simulink model "voltage_to_fahrenheit_system"  (R2020b)
settings: Solver=ode45  StartTime=0.0  StopTime=220  RelTol=1e-3  EnableMultiTasking=on
libraries: simulink x1
settings Model: Creator=USER  LastModifiedBy=USER
settings DataIOCC: LimitDataPoints=on  SaveFormat=Array  ReturnWorkspaceOutputs=off
settings OptimizationCC: LifeSpan=inf
settings DebuggingCC: SFUnexpectedBacktrackingDiag=warning  SFNoUnconditionalDefaultTransitionDiag=warning  SFExecutionAtInitializationDiag=none  ArithmeticOperatorsInVariantConditions=warning
settings HardwareCC: ProdBitPerPointer=32  ProdBitPerSizeT=32  ProdBitPerPtrDiffT=32  ProdLargestAtomicFloat=None  ProdIntDivRoundTo=Undefined  ProdEndianess=Unspecified  ProdWordSize=32  ProdHWDeviceType=32-bit Generic
settings ModelReferenceCC: PropagateSignalLabelsOutOfModel=off
settings SFSimCC: SimUseLocalCustomCode=off  CustomCodeUndefinedFunction=UseInterfaceOnly
settings RTWCC: RTWUseLocalCustomCode=off
settings CodeAppCC: StateflowObjectComments=on
settings GRTTargetCC: TargetLangStandard=C89/C90 (ANSI)
settings ConfigComp: CovMetricSettings=dw  CovSaveCumulativeToWorkspaceVar=on  CovSaveSingleToWorkspaceVar=on  CovExternalEMLEnable=off

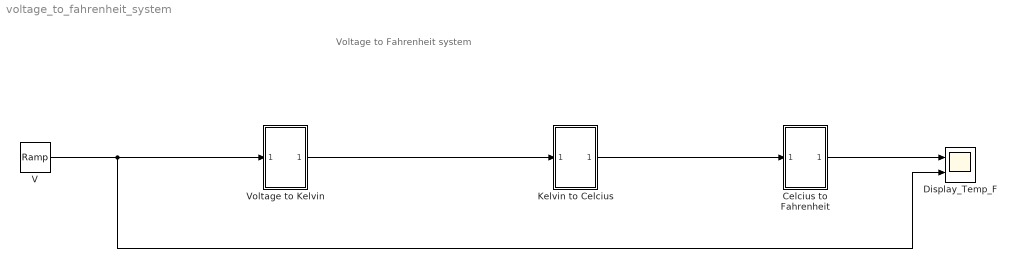
== system voltage_to_fahrenheit_system ==
  note: Voltage to Fahrenheit system
  Celcius to Fahrenheit : Subsystem
  Display_Temp_F : Scope  NumInputPorts=2
  Kelvin to Celcius : Subsystem
  V : simulink/Sources/Ramp  slope=20  start=0  InitialOutput=0
  Voltage to Kelvin : Subsystem
  wires:
  V/1 -> Display_Temp_F/2, Voltage to Kelvin/1(In1)
  Voltage to Kelvin/1(Out1) -> Kelvin to Celcius/1(In1)
  Kelvin to Celcius/1(Out1) -> Celcius to Fahrenheit/1(In1)
  Celcius to Fahrenheit/1(Out1) -> Display_Temp_F/1

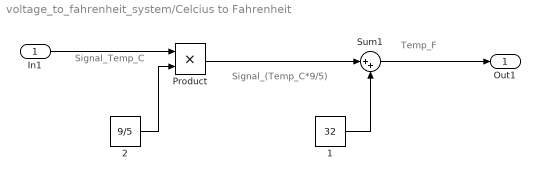
== system voltage_to_fahrenheit_system/Celcius to Fahrenheit ==
  note: Temp_F
  note: Signal_(Temp_C*9/5)
  note: Signal_Temp_C
  In1 : Inport
  " 1" : Constant  Value=32
  " 2" : Constant  Value=9/5
  Product : Product
  Sum1 : Sum  Inputs=|++
  Out1 : Outport
  wires:
  " 2"/1 -> Product/2
  Product/1 -> Sum1/1
  In1/1 -> Product/1
  Sum1/1 -> Out1/1
  " 1"/1 -> Sum1/2

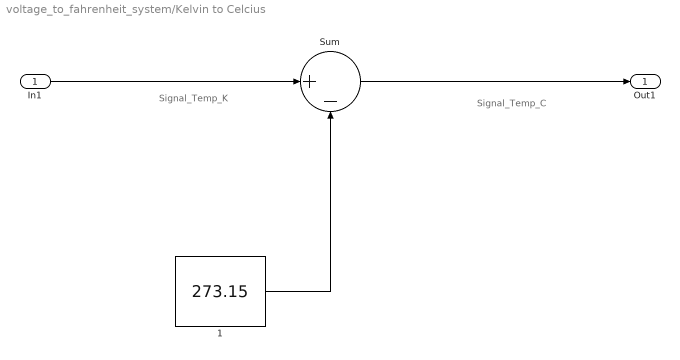
== system voltage_to_fahrenheit_system/Kelvin to Celcius ==
  note: Signal_Temp_C
  note: Signal_Temp_K
  In1 : Inport
  " 1" : Constant  Value=273.15
  Sum : Sum  Inputs=|+-
  Out1 : Outport
  wires:
  " 1"/1 -> Sum/2
  In1/1 -> Sum/1
  Sum/1 -> Out1/1

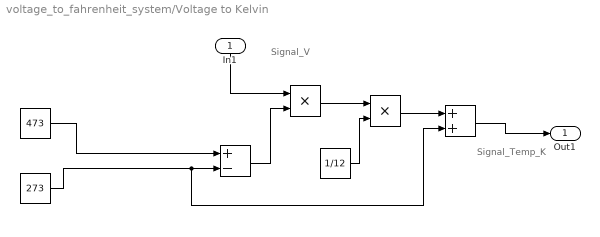
== system voltage_to_fahrenheit_system/Voltage to Kelvin ==
  note: Signal_V
  note: Signal_Temp_K
  In1 : Inport
  " " : Constant  Value=473
  "  " : Constant  Value=273
  "   " : Constant  Value=1/12
  "    " : Product
  "     " : Sum  Inputs=+-
  "      " : Sum
  "       " : Product
  Out1 : Outport
  wires:
  "   "/1 -> "       "/2
  "      "/1 -> Out1/1
  "  "/1 -> "      "/2, "     "/2
  "     "/1 -> "    "/2
  "    "/1 -> "       "/1
  "       "/1 -> "      "/1
  " "/1 -> "     "/1
  In1/1 -> "    "/1
